simulink library "HEV_Battery_Lib_org"  (Simulink 10.0)
settings: Solver=ode45  StartTime=0.0  StopTime=10.0  RelTol=1e-3  EnableMultiTasking=on
undefined symbols (not defined in the file): HEV_Param, Hydride, Kt_Temps, Metal, Nickel
libraries: fl_lib x55, nesl_utility x30, LeadAcidBattery_lib x12, $bdroot x9, fl_ps_legacy_lib x9, ee_lib x3, powerlib x3, Capacitors_lib x1, electricdrivelib x1
Description:
  | Copyright 2014-2017 The MathWorks, Inc.
settings Model: Creator=smiller  LastModifiedBy=annonymous

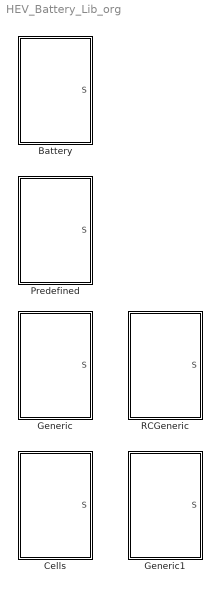
== system HEV_Battery_Lib_org ==
  Battery : Subsystem  BlockChoice=Generic
      settings: TemplateBlock=self  MemberBlocks=Cells,Generic,Predefined
      mask Display: disp(' ')
  Cells : Subsystem
      mask Display:
      | image(imread('HEV_Battery_Cells_IMAGE.jpg'));
      | port_label('LConn',1,'+');
      | port_label('LConn',2,'-');
      | port_label('output',1,'S');
  Generic : Subsystem
      mask Display:
      | image(imread('HEV_Battery_Custom_IMAGE.jpg'));
      | port_label('LConn',1,'+');
      | port_label('LConn',2,'-');
      | port_label('output',1,'S');
  Generic1 : Subsystem
      mask Display:
      | image(imread('HEV_Battery_Generic_IMAGE.jpg'));
      | port_label('LConn',1,'+');
      | port_label('LConn',2,'-');
      | port_label('output',1,'S');
  Predefined : Subsystem
      mask Display:
      | image(imread('HEV_Battery_Detailed_IMAGE.jpg'));
      | port_label('LConn',1,'+');
      | port_label('LConn',2,'-');
      | port_label('output',1,'S');
  RCGeneric : Subsystem
      mask Display:
      | image(imread('HEV_Battery_GenericRC_IMAGE.jpg'));
      | port_label('LConn',1,'+');
      | port_label('LConn',2,'-');
      | port_label('output',1,'S');

== system HEV_Battery_Lib_org/Battery ==
  Generic : $bdroot/Generic  SystemSampleTime=-1  Latency=0  AutoFrameSizeCalculation=off
  + : PMIOPort  Side=Left
  - : PMIOPort  Port=2  Side=Left
  S : Outport
  wires:
  Generic/1 -> S/1
  connections:
  Generic/LConn1 -- +/RConn1
  Generic/LConn2 -- -/RConn1

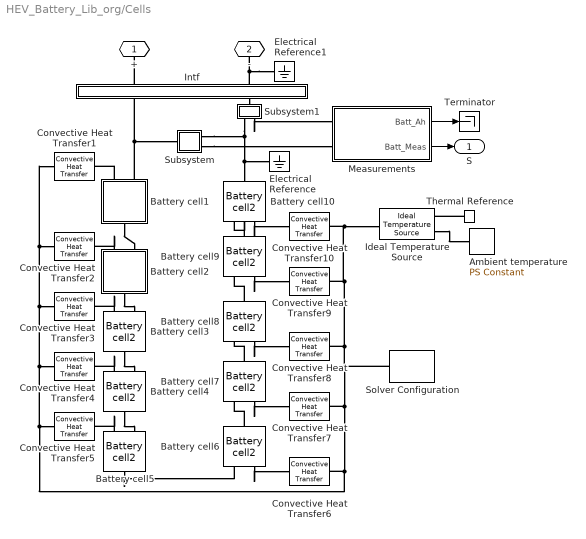
== system HEV_Battery_Lib_org/Cells ==
  Ambient temperature : fl_lib/Physical Signals/Sources/PS Constant  constant=273+25
  Battery cell1 : Subsystem
      mask Display:
      | % Battery icon
      | plot([1.5 0.4],[0 0])
      | plot(-[0.2 0.9 0.9 1.5],[0 0 -0.8 -0.8])
      | patch(([1 1 -1 -1]*0.15-0.5)*-1,[-1 1 1 -1]*0.4,[0;0;0]);
      | patch(([1 1 -1 -1]*0.15+0.1)*-1,[-1 1 1 -1]*0.9,[0;0;0]);
      | 
      | % Thermal port
      | plot([-0.5,-0.9],[1.2,1.2])
      | plot([-0.5,-0.9],[0.4,0.4])
      | plot([-0.9,-1.5],[0.8,0.8])
      | plot(-0.15*sin(0:2*pi/50:2*pi)-0.85,-0.35*cos(0:2*pi/50:2*pi)+0.8)
      | plot(0.15*sin(0:2*pi/50:pi)-0.55,-0.35*cos(0:2*pi/50:pi)+0.8)
      | 
      | % Plot points to set plot range
      | color('white');plot(1.5,1.5);plot(-1.5,-1.5)
      | 
      | color('red')
      | port_label('LConn',1,'H')
      | port_label('LConn',2,'+')
      | port_label('RConn',1,'-')
  Battery cell{3..10} (8 alike) : $bdroot/Cells/Battery cell2  SystemSampleTime=-1
  Battery cell2 : Subsystem
      mask Display:
      | % Battery icon
      | plot([1.5 0.4],[0 0])
      | plot(-[0.2 0.9 0.9 1.5],[0 0 -0.8 -0.8])
      | patch(([1 1 -1 -1]*0.15-0.5)*-1,[-1 1 1 -1]*0.4,[0;0;0]);
      | patch(([1 1 -1 -1]*0.15+0.1)*-1,[-1 1 1 -1]*0.9,[0;0;0]);
      | 
      | % Thermal port
      | plot([-0.5,-0.9],[1.2,1.2])
      | plot([-0.5,-0.9],[0.4,0.4])
      | plot([-0.9,-1.5],[0.8,0.8])
      | plot(-0.15*sin(0:2*pi/50:2*pi)-0.85,-0.35*cos(0:2*pi/50:2*pi)+0.8)
      | plot(0.15*sin(0:2*pi/50:pi)-0.55,-0.35*cos(0:2*pi/50:pi)+0.8)
      | 
      | % Plot points to set plot range
      | color('white');plot(1.5,1.5);plot(-1.5,-1.5)
      | 
      | color('red')
      | port_label('LConn',1,'H')
      | port_label('LConn',2,'+')
      | port_label('RConn',1,'-')
  Convective Heat Transfer{1..10} (10 alike) : fl_lib/Thermal/Thermal Elements/Convective Heat Transfer  area=HEV_Param.Battery_Cell.Area m^2  heat_tr_coeff=HEV_Param.Battery_Cell.Rtheta W/(m^2 *K)  Q_specify=off  Q_priority=High  Q=0 J/s  Q_nominal_specify=off  Q_nominal_unit=J/s  Q_nominal_value=1  T_specify=off  T_priority=High  T=0 K  T_nominal_specify=off  T_nominal_unit=K  T_nominal_value=1
  Electrical Reference : fl_lib/Electrical/Electrical Elements/Electrical Reference
  Electrical Reference1 : fl_lib/Electrical/Electrical Elements/Electrical Reference
  Ideal Temperature Source : fl_lib/Thermal/Thermal Sources/Ideal Temperature Source
      settings: SourceProductName=Simscape  SourceProductBaseCode=SS
  Intf : Subsystem  mask(Simscape Interface Element){T=100000}
      mask prompts: T "Pole in Transfer Function"
      mask help:
      | Ideal transformer between Simscape circuits.
      |
      | The Voltage across the two terminal pairs are equal and the current flowing through the two branches are equal.
      |
      | The coupling has a transfer function and you need to set the pole in the transfer function.
      mask Display:
      | %color('red');
      | %plot([0.3 0.7],[0.775 0.775]);
      | port_label('LConn', 1,'SPS1')
      | port_label('RConn', 1,'SS1')
      | color('black');
      | %plot([0.3 0.7],[0.225 0.225]);
      | port_label('LConn', 2,'SPS2')
      | port_label('RConn', 2,'SS2')
      | color('green')
      | %text(0.05,0.5,'I Src');
      | color('blue')
      | %text(0.75,0.5,'V Src');
  Measurements : Subsystem
  Solver Configuration : nesl_utility/Solver Configuration  PhysicalDomain=network_engine_domain  SubClassName=solver  LeftPortType=input  RightPortType=generic  Accelerate=off  Tones=[]  Harmonics=[]  SimulateNoise=off  Profile=off  UseLocalSampling=off  EnableSwitchedLinearOptims=on  FrequencyDomain=off  UseCCode=off  RelTol=0.001  AbsTol=1e-06  MinStep=1e-09  ToWorkspace=off  RevertToSquareIcSolve=off  NumHomotopyIterations=100  PhasorMode=off  PhasorModeNumHarmonics=1  OverrideAbsTol=off  DoDC=off  ResidualTolerance=1e-9  UseLocalSolver=off  LocalSolverChoice=NE_BACKWARD_EULER_ADVANCER  LocalSolverSampleTime=.001  DoFixedCost=off  MaxNonlinIter=3  MaxModeIter=2  LinearAlgebra=Sparse  DelaysMemoryBudget=1024  AutomaticFiltering=on  FilteringTimeConstant=0.001
  Subsystem : Subsystem
      mask Display: disp('S')
  Subsystem1 : Subsystem
      mask Display: disp('S');
  Terminator : Terminator
  Thermal Reference : fl_lib/Thermal/Thermal Elements/Thermal Reference
  + : PMIOPort  Side=Left
  - : PMIOPort  Port=2  Side=Left
  S : Outport
  wires:
  Measurements/2(Batt_Meas) -> S/1
  Measurements/1(Batt_Ah) -> Terminator/1
  connections:
  Electrical Reference1/LConn1 -- -/RConn1 -- Intf/RConn2
  Intf/RConn1 -- +/RConn1
  Intf/LConn2 -- Subsystem1/LConn1
  Subsystem1/RConn2 -- Measurements/LConn1
  Subsystem1/RConn1 -- Battery cell10/RConn1 -- Electrical Reference/LConn1 -- Subsystem/RConn2
  Subsystem/RConn1 -- Measurements/LConn2
  Convective Heat Transfer6/LConn1 -- Convective Heat Transfer1/LConn1 -- Convective Heat Transfer2/LConn1 -- Convective Heat Transfer3/LConn1 -- Convective Heat Transfer4/LConn1 -- Convective Heat Transfer5/LConn1 -- Solver Configuration/RConn1 -- Convective Heat Transfer8/LConn1 -- Convective Heat Transfer10/LConn1 -- Ideal Temperature Source/LConn1 -- Convective Heat Transfer9/LConn1 -- Convective Heat Transfer7/LConn1
  Battery cell1/LConn2 -- Subsystem/LConn1 -- Intf/LConn1
  Battery cell9/LConn1 -- Convective Heat Transfer9/RConn1
  Battery cell8/RConn1 -- Battery cell9/LConn2
  Battery cell8/LConn1 -- Convective Heat Transfer8/RConn1
  Battery cell7/LConn1 -- Convective Heat Transfer7/RConn1
  Battery cell7/RConn1 -- Battery cell8/LConn2
  Battery cell6/LConn1 -- Convective Heat Transfer6/RConn1
  Battery cell6/RConn1 -- Battery cell7/LConn2
  Battery cell5/RConn1 -- Battery cell6/LConn2
  Battery cell5/LConn1 -- Convective Heat Transfer5/RConn1
  Battery cell4/RConn1 -- Battery cell5/LConn2
  Battery cell4/LConn1 -- Convective Heat Transfer4/RConn1
  Battery cell3/RConn1 -- Battery cell4/LConn2
  Battery cell3/LConn1 -- Convective Heat Transfer3/RConn1
  Battery cell2/RConn1 -- Battery cell3/LConn2
  Battery cell9/RConn1 -- Battery cell10/LConn2
  Battery cell2/LConn1 -- Convective Heat Transfer2/RConn1
  Battery cell10/LConn1 -- Convective Heat Transfer10/RConn1
  Battery cell1/RConn1 -- Battery cell2/LConn2
  Battery cell1/LConn1 -- Convective Heat Transfer1/RConn1
  Ideal Temperature Source/RConn1 -- Ambient temperature/RConn1
  Thermal Reference/LConn1 -- Ideal Temperature Source/RConn2

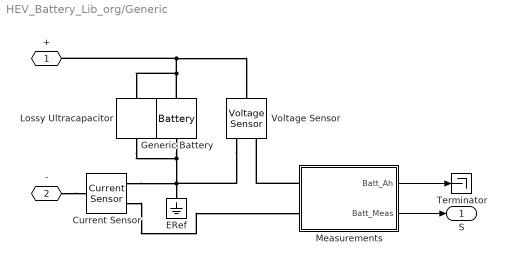
== system HEV_Battery_Lib_org/Generic ==
  Current Sensor : fl_lib/Electrical/Electrical Sensors/Current Sensor
  ERef : fl_lib/Electrical/Electrical Elements/Electrical Reference
  Generic Battery : ee_lib/Sources/Battery  Vnom=HEV_Param.Battery_Sys.Nominal_Voltage V  R1=HEV_Param.Battery_Sys.Internal_Resistance Ohm  prm_AH=2  AH=HEV_Param.Battery_Sys.Rated_Capacity hr*A  V1=HEV_Param.Battery_Sys.Expn_Voltage V  AH1=HEV_Param.Battery_Sys.Expn_Charge hr*A  prm_R2=1  R2=2e+3 Ohm  prm_dyn=1  Rp1=0.005 Ohm  tau1=30 s  Rp2=0.005 Ohm  tau2=30 s  Rp3=0.005 Ohm  tau3=30 s  Rp4=0.005 Ohm  tau4=30 s  Rp5=0.005 Ohm  tau5=30 s  prm_fade=1  N_fade=100  AH_fade=45 hr*A  R1_fade=2.02 Ohm  V1_fade=10.35 V  i_specify=off  i_priority=None  i=0 A  i_nominal_specify=off  i_nominal_unit=A  i_nominal_value=1  v_specify=off  v_priority=None  v=0 V  v_nominal_specify=off  v_nominal_unit=V  v_nominal_value=1  charge_specify=on  charge_priority=High  charge=HEV_Param.Battery_Sys.Initial_Charge hr*A  charge_nominal_specify=off  charge_nominal_unit=hr*A  charge_nominal_value=1  num_cycles_specify=off  num_cycles_priority=High  num_cycles=0  num_cycles_nominal_specify=off  num_cycles_nominal_unit=1  num_cycles_nominal_value=1  thermal_mass=30000 J/K  Tmeas=298.15 K  Vnom_T2=12 V  R1_T2=2.2 Ohm  V1_T2=11.4 V  R2_T2=2200 Ohm  Rp1_T2=0.005 Ohm  tau1_T2=30 s  Rp2_T2=0.005 Ohm  tau2_T2=30 s  Rp3_T2=0.005 Ohm  tau3_T2=30 s  Rp4_T2=0.005 Ohm  tau4_T2=30 s  Rp5_T2=0.005 Ohm  tau5_T2=30 s  Tmeas2=273.15 K  temperature_specify=off  temperature_priority=High  temperature=298.15 K  temperature_nominal_specify=off  temperature_nominal_unit=K  temperature_nominal_value=1
      settings: SourceProductName=Simscape Electrical
  Lossy Ultracapacitor : Capacitors_lib/Lossy Ultracapacitor  C0=HEV_Param.UltraCapacitor.Nominal_Capacitance F  Cv=HEV_Param.UltraCapacitor.Rate_C_V F/V  R=HEV_Param.UltraCapacitor.Series_R Ohm  Rd=HEV_Param.UltraCapacitor.Self_Discharge_R Ohm  i_specify=off  i_priority=High  i=0 A  i_nominal_specify=off  i_nominal_unit=A  i_nominal_value=1  vc_specify=off  vc_priority=High  vc=0 V  vc_nominal_specify=off  vc_nominal_unit=V  vc_nominal_value=1
      settings: InternalSimscapePortConfiguration="{\"Bottom\":[],\"Left\":[{\"id\":\"p\",\"label\":\"+\",\"type\":\"foundation.electrical.electrical\"}],\"Right\":[{\"id\":\"n\",\"label\":\"-\",\"type\":\"foundation.electrical.electrical\"}],\"Top\":[]}"
  Measurements : Subsystem
  Terminator : Terminator
  Voltage Sensor : fl_lib/Electrical/Electrical Sensors/Voltage Sensor
  + : PMIOPort  Side=Left
  - : PMIOPort  Port=2  Side=Left
  S : Outport
  wires:
  Measurements/1(Batt_Ah) -> Terminator/1
  Measurements/2(Batt_Meas) -> S/1
  connections:
  Measurements/LConn1 -- Voltage Sensor/RConn1
  Generic Battery/LConn1 -- Voltage Sensor/LConn1 -- +/RConn1 -- Lossy Ultracapacitor/LConn1
  Generic Battery/RConn1 -- Voltage Sensor/RConn2 -- ERef/LConn1 -- Current Sensor/RConn2 -- Lossy Ultracapacitor/RConn1
  Current Sensor/RConn1 -- Measurements/LConn2
  -/RConn1 -- Current Sensor/LConn1

== system HEV_Battery_Lib_org/Generic1 ==
  Current Sensor : fl_lib/Electrical/Electrical Sensors/Current Sensor
  Electrical Reference : fl_lib/Electrical/Electrical Elements/Electrical Reference
  Generic Battery : ee_lib/Sources/Battery  Vnom=HEV_Param.Battery_Sys.Nominal_Voltage V  R1=HEV_Param.Battery_Sys.Internal_Resistance Ohm  prm_AH=2  AH=HEV_Param.Battery_Sys.Rated_Capacity hr*A  V1=HEV_Param.Battery_Sys.Expn_Voltage V  AH1=HEV_Param.Battery_Sys.Expn_Charge hr*A  prm_R2=1  R2=2e+3 Ohm  prm_dyn=1  Rp1=0.005 Ohm  tau1=30 s  Rp2=0.005 Ohm  tau2=30 s  Rp3=0.005 Ohm  tau3=30 s  Rp4=0.005 Ohm  tau4=30 s  Rp5=0.005 Ohm  tau5=30 s  prm_fade=1  N_fade=100  AH_fade=45 hr*A  R1_fade=2.02 Ohm  V1_fade=10.35 V  i_specify=off  i_priority=None  i=0 A  i_nominal_specify=off  i_nominal_unit=A  i_nominal_value=1  v_specify=off  v_priority=None  v=0 V  v_nominal_specify=off  v_nominal_unit=V  v_nominal_value=1  charge_specify=on  charge_priority=High  charge=HEV_Param.Battery_Sys.Initial_Charge hr*A  charge_nominal_specify=off  charge_nominal_unit=hr*A  charge_nominal_value=1  num_cycles_specify=off  num_cycles_priority=High  num_cycles=0  num_cycles_nominal_specify=off  num_cycles_nominal_unit=1  num_cycles_nominal_value=1  thermal_mass=30000 J/K  Tmeas=298.15 K  Vnom_T2=12 V  R1_T2=2.2 Ohm  V1_T2=11.4 V  R2_T2=2200 Ohm  Rp1_T2=0.005 Ohm  tau1_T2=30 s  Rp2_T2=0.005 Ohm  tau2_T2=30 s  Rp3_T2=0.005 Ohm  tau3_T2=30 s  Rp4_T2=0.005 Ohm  tau4_T2=30 s  Rp5_T2=0.005 Ohm  tau5_T2=30 s  Tmeas2=273.15 K  temperature_specify=off  temperature_priority=High  temperature=298.15 K  temperature_nominal_specify=off  temperature_nominal_unit=K  temperature_nominal_value=1
      settings: SourceProductName=Simscape Electrical
  Measurements : Subsystem
  Terminator : Terminator
  Voltage Sensor1 : fl_lib/Electrical/Electrical Sensors/Voltage Sensor
  + : PMIOPort  Side=Left
  - : PMIOPort  Port=2  Side=Left
  S : Outport
  wires:
  Measurements/2(Batt_Meas) -> S/1
  Measurements/1(Batt_Ah) -> Terminator/1
  connections:
  -/RConn1 -- Current Sensor/LConn1
  Current Sensor/RConn1 -- Measurements/LConn2
  Current Sensor/RConn2 -- Electrical Reference/LConn1 -- Generic Battery/RConn1 -- Voltage Sensor1/RConn2
  +/RConn1 -- Generic Battery/LConn1 -- Voltage Sensor1/LConn1
  Measurements/LConn1 -- Voltage Sensor1/RConn1

== system HEV_Battery_Lib_org/Predefined ==
  Electrical Reference : fl_lib/Electrical/Electrical Elements/Electrical Reference
  GF1 : Subsystem
      mask Display: disp('GF')
  Ground : powerlib/Elements/Ground  LConnTagsString=a
      settings: SourceProductName=Simscape Electrical
  Intf : Subsystem  mask(Power Systems ST - Simscape Interface Element){T=100000}
      mask prompts: T "Pole in Transfer Function"
      mask help:
      | Ideal transformer between a Simscape Power Systems ST circuit and a Simscape circuit.
      |
      | The Voltage across the two terminal pairs are equal and the current flowing through the two branches are equal.
      |
      | The coupling has a transfer function and you need to set the pole in the transfer function.
      mask Display:
      | %color('red');
      | %plot([0.3 0.7],[0.775 0.775]);
      | port_label('LConn', 1,'SPS1')
      | port_label('RConn', 1,'SS1')
      | color('black');
      | %plot([0.3 0.7],[0.225 0.225]);
      | port_label('LConn', 2,'SPS2')
      | port_label('RConn', 2,'SS2')
      | color('green')
      | %text(0.05,0.5,'I Src');
      | color('blue')
      | %text(0.75,0.5,'V Src');
  Preset Battery : electricdrivelib/Extra Sources/Battery  BatType=Nickel-Metal-Hydride  ShowTempParam=off  ThermalPreset=no  ShowAgeParam=off  NomV=HEV_Param.Battery_Det.Nominal_Voltage  NomQ=HEV_Param.Battery_Det.Rated_Capacity  SOC=HEV_Param.Battery_Det.Initial_SOC  Batt_Tr=30  PresetModel=on  MaxQ=8.7231  MinV=150  FullV=235.5932  Dis_rate=1.62  R=0.24691  Normal_OP=7.7885  expZone="[216.9492          1.62]"  current=[50 100]  Units=Time  Tci=20  NomT=20  T2=-30  MaxQ2=4.8  FullV2=7.1  Normal_OP2=5.72  expZone2="[6.58  1]"  Rca=0.6  ti=1000  Dp=0  Neq0=0  Tsim=1e6  Ta1=25  Qeol=5.4*0.9  Reol=0.013333*1.2  Char_age=[2.3478, 3]  Dis_age=[2.3478, 10]  N1=1500  N2=10500  N3=1000  N4=1400  Ta2=45  N5=950
      settings: SourceProductName=Simscape Electrical
  + : PMIOPort  Side=Left
  - : PMIOPort  Port=2  Side=Left
  S : Outport
  wires:
  Preset Battery/1 -> GF1/1(In1)
  GF1/1(Out1) -> S/1
  connections:
  Intf/RConn2 -- Electrical Reference/LConn1 -- -/RConn1
  Intf/LConn2 -- Ground/LConn1 -- Preset Battery/LConn2
  Preset Battery/LConn1 -- Intf/LConn1
  +/RConn1 -- Intf/RConn1

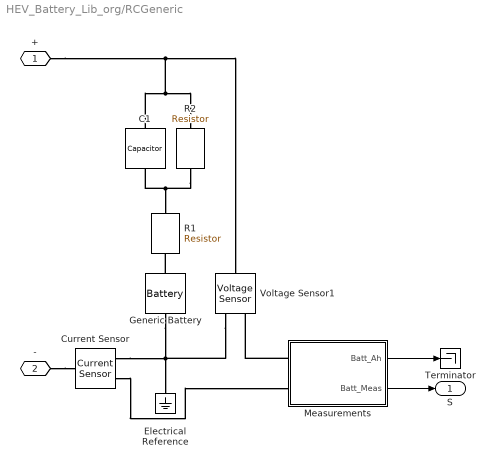
== system HEV_Battery_Lib_org/RCGeneric ==
  C1 : fl_lib/Electrical/Electrical Elements/Capacitor  c=HEV_Param.Battery_Sys.C1.Capacitance F  r=HEV_Param.Battery_Sys.C1.Series_Resistance Ohm  g=0 1/Ohm  i_specify=off  i_priority=High  i=0 A  i_nominal_specify=off  i_nominal_unit=A  i_nominal_value=1  v_specify=off  v_priority=High  v=0 V  v_nominal_specify=off  v_nominal_unit=V  v_nominal_value=1  vc_specify=on  vc_priority=High  vc=HEV_Param.Battery_Sys.C1.Initial_Voltage V  vc_nominal_specify=off  vc_nominal_unit=V  vc_nominal_value=1
  Current Sensor : fl_lib/Electrical/Electrical Sensors/Current Sensor
  Electrical Reference : fl_lib/Electrical/Electrical Elements/Electrical Reference
  Generic Battery : ee_lib/Sources/Battery  Vnom=HEV_Param.Battery_Sys.Nominal_Voltage V  R1=HEV_Param.Battery_Sys.Internal_Resistance Ohm  prm_AH=2  AH=HEV_Param.Battery_Sys.Rated_Capacity hr*A  V1=HEV_Param.Battery_Sys.Expn_Voltage V  AH1=HEV_Param.Battery_Sys.Expn_Charge hr*A  prm_R2=1  R2=2e+3 Ohm  prm_dyn=1  Rp1=0.005 Ohm  tau1=30 s  Rp2=0.005 Ohm  tau2=30 s  Rp3=0.005 Ohm  tau3=30 s  Rp4=0.005 Ohm  tau4=30 s  Rp5=0.005 Ohm  tau5=30 s  prm_fade=1  N_fade=100  AH_fade=45 hr*A  R1_fade=2.02 Ohm  V1_fade=10.35 V  i_specify=off  i_priority=None  i=0 A  i_nominal_specify=off  i_nominal_unit=A  i_nominal_value=1  v_specify=off  v_priority=None  v=0 V  v_nominal_specify=off  v_nominal_unit=V  v_nominal_value=1  charge_specify=on  charge_priority=High  charge=HEV_Param.Battery_Sys.Initial_Charge hr*A  charge_nominal_specify=off  charge_nominal_unit=hr*A  charge_nominal_value=1  num_cycles_specify=off  num_cycles_priority=High  num_cycles=0  num_cycles_nominal_specify=off  num_cycles_nominal_unit=1  num_cycles_nominal_value=1  thermal_mass=30000 J/K  Tmeas=298.15 K  Vnom_T2=12 V  R1_T2=2.2 Ohm  V1_T2=11.4 V  R2_T2=2200 Ohm  Rp1_T2=0.005 Ohm  tau1_T2=30 s  Rp2_T2=0.005 Ohm  tau2_T2=30 s  Rp3_T2=0.005 Ohm  tau3_T2=30 s  Rp4_T2=0.005 Ohm  tau4_T2=30 s  Rp5_T2=0.005 Ohm  tau5_T2=30 s  Tmeas2=273.15 K  temperature_specify=off  temperature_priority=High  temperature=298.15 K  temperature_nominal_specify=off  temperature_nominal_unit=K  temperature_nominal_value=1
      settings: SourceProductName=Simscape Electrical
  Measurements : Subsystem
  R1 : fl_lib/Electrical/Electrical Elements/Resistor  R=HEV_Param.Battery_Sys.R1 Ohm  i_specify=off  i_priority=High  i=0 A  i_nominal_specify=off  i_nominal_unit=A  i_nominal_value=1  v_specify=off  v_priority=High  v=0 V  v_nominal_specify=off  v_nominal_unit=V  v_nominal_value=1
  R2 : fl_lib/Electrical/Electrical Elements/Resistor  R=HEV_Param.Battery_Sys.R2 Ohm  i_specify=off  i_priority=High  i=0 A  i_nominal_specify=off  i_nominal_unit=A  i_nominal_value=1  v_specify=off  v_priority=High  v=0 V  v_nominal_specify=off  v_nominal_unit=V  v_nominal_value=1
  Terminator : Terminator
  Voltage Sensor1 : fl_lib/Electrical/Electrical Sensors/Voltage Sensor
  + : PMIOPort  Side=Left
  - : PMIOPort  Port=2  Side=Left
  S : Outport
  wires:
  Measurements/1(Batt_Ah) -> Terminator/1
  Measurements/2(Batt_Meas) -> S/1
  connections:
  Measurements/LConn1 -- Voltage Sensor1/RConn1
  +/RConn1 -- Voltage Sensor1/LConn1 -- R2/LConn1 -- C1/LConn1
  Voltage Sensor1/RConn2 -- Generic Battery/RConn1 -- Electrical Reference/LConn1 -- Current Sensor/RConn2
  Current Sensor/RConn1 -- Measurements/LConn2
  -/RConn1 -- Current Sensor/LConn1
  R2/RConn1 -- R1/LConn1 -- C1/RConn1
  Generic Battery/LConn1 -- R1/RConn1

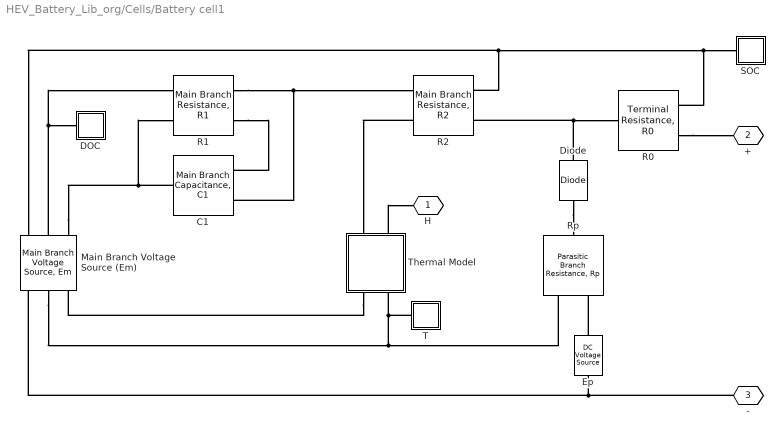
== system HEV_Battery_Lib_org/Cells/Battery cell1 ==
  " DOC " : Subsystem
  " SOC " : Subsystem
  C1 : LeadAcidBattery_lib/Main Branch Capacitance, C1  Tau1=HEV_Param.Battery_Cell.Tau1 s  Cmin=1e-5 F
  Diode : fl_lib/Electrical/Electrical Elements/Diode  Vf=0.6 V  Ron=0.3 Ohm  Goff=1e-08 1/Ohm  i_specify=off  i_priority=High  i=0 A  i_nominal_specify=off  i_nominal_unit=A  i_nominal_value=1  v_specify=off  v_priority=High  v=0 V  v_nominal_specify=off  v_nominal_unit=V  v_nominal_value=1
  Ep : fl_lib/Electrical/Electrical Sources/DC Voltage Source  v0=HEV_Param.Battery_Cell.Ep V
  Main Branch Voltage Source (Em) : LeadAcidBattery_lib/Main Branch Voltage Source, Em  Em0=HEV_Param.Battery_Cell.Emo V  Ke=HEV_Param.Battery_Cell.Ke V/K  Kc=HEV_Param.Battery_Cell.Kc  C0=HEV_Param.Battery_Cell.Costar s*A  Istar=HEV_Param.Battery_Cell.Istar A  delta=HEV_Param.Battery_Cell.delta  Tau1=HEV_Param.Battery_Cell.Tau1 s  Qinit=HEV_Param.Battery_Cell.Qe_init s*A
  R0 : LeadAcidBattery_lib/Terminal Resistance, R0  R00=HEV_Param.Battery_Cell.Roo Ohm  A0=HEV_Param.Battery_Cell.Ao
  R1 : LeadAcidBattery_lib/Main Branch Resistance, R1  R10=HEV_Param.Battery_Cell.R10 Ohm  DOC_min=1e-006
  R2 : LeadAcidBattery_lib/Main Branch Resistance, R2  R20=HEV_Param.Battery_Cell.R20 Ohm  A21=HEV_Param.Battery_Cell.A21  A22=HEV_Param.Battery_Cell.A22  Istar=HEV_Param.Battery_Cell.Istar A
  Rp : LeadAcidBattery_lib/Parasitic Branch Resistance, Rp  Gp0=HEV_Param.Battery_Cell.Gpo 1/Ohm  Vp0=HEV_Param.Battery_Cell.Vpo V  Ap=HEV_Param.Battery_Cell.Ap  Tf=HEV_Param.Battery_Cell.theta_f degC
  T : Subsystem
  Thermal Model : Subsystem
  H : PMIOPort  Tag=PMCPort  Side=Left
  + : PMIOPort  Tag=PMCPort  Port=2  Side=Left
  - : PMIOPort  Tag=PMCPort  Port=3  Side=Right
  connections:
  Diode/LConn1 -- R0/RConn1 -- R2/LConn2
  R2/RConn2 -- Thermal Model/LConn1
  -/RConn1 -- Ep/RConn1 -- Main Branch Voltage Source (Em)/RConn1
  Thermal Model/RConn1 -- Main Branch Voltage Source (Em)/RConn3
  Diode/RConn1 -- Rp/LConn1
  Ep/LConn1 -- Rp/RConn2
  Thermal Model/LConn2 -- H/RConn1
  R2/LConn1 -- Main Branch Voltage Source (Em)/LConn1 -- R0/LConn1 -- " SOC "/LConn1
  R1/LConn2 -- C1/LConn1
  R1/LConn1 -- C1/LConn2 -- R2/RConn1
  Main Branch Voltage Source (Em)/LConn3 -- C1/RConn1 -- R1/RConn2
  Main Branch Voltage Source (Em)/LConn2 -- R1/RConn1 -- " DOC "/LConn1
  R0/LConn2 -- +/RConn1
  Main Branch Voltage Source (Em)/RConn2 -- Rp/RConn1 -- T/LConn1 -- Thermal Model/RConn2

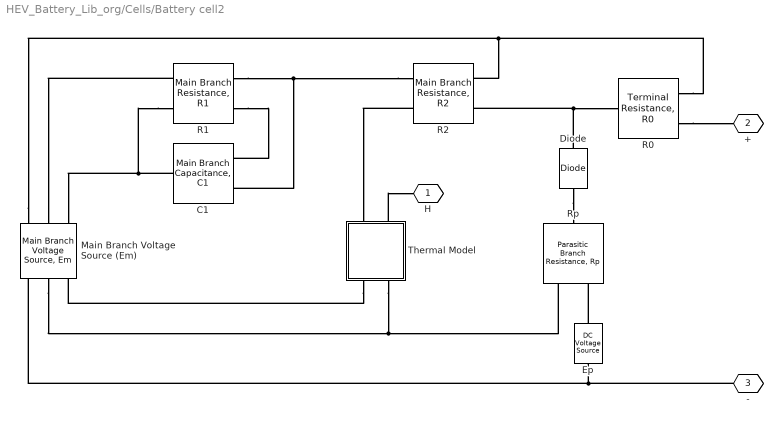
== system HEV_Battery_Lib_org/Cells/Battery cell2 ==
  C1 : LeadAcidBattery_lib/Main Branch Capacitance, C1  Tau1=HEV_Param.Battery_Cell.Tau1 s  Cmin=1e-5 F
  Diode : fl_lib/Electrical/Electrical Elements/Diode  Vf=0.6 V  Ron=0.3 Ohm  Goff=1e-08 1/Ohm  i_specify=off  i_priority=High  i=0 A  i_nominal_specify=off  i_nominal_unit=A  i_nominal_value=1  v_specify=off  v_priority=High  v=0 V  v_nominal_specify=off  v_nominal_unit=V  v_nominal_value=1
  Ep : fl_lib/Electrical/Electrical Sources/DC Voltage Source  v0=HEV_Param.Battery_Cell.Ep V
  Main Branch Voltage Source (Em) : LeadAcidBattery_lib/Main Branch Voltage Source, Em  Em0=HEV_Param.Battery_Cell.Emo V  Ke=HEV_Param.Battery_Cell.Ke V/K  Kc=HEV_Param.Battery_Cell.Kc  C0=HEV_Param.Battery_Cell.Costar s*A  Istar=HEV_Param.Battery_Cell.Istar A  delta=HEV_Param.Battery_Cell.delta  Tau1=HEV_Param.Battery_Cell.Tau1 s  Qinit=HEV_Param.Battery_Cell.Qe_init s*A
  R0 : LeadAcidBattery_lib/Terminal Resistance, R0  R00=HEV_Param.Battery_Cell.Roo Ohm  A0=HEV_Param.Battery_Cell.Ao
  R1 : LeadAcidBattery_lib/Main Branch Resistance, R1  R10=HEV_Param.Battery_Cell.R10 Ohm  DOC_min=1e-006
  R2 : LeadAcidBattery_lib/Main Branch Resistance, R2  R20=HEV_Param.Battery_Cell.R20 Ohm  A21=HEV_Param.Battery_Cell.A21  A22=HEV_Param.Battery_Cell.A22  Istar=HEV_Param.Battery_Cell.Istar A
  Rp : LeadAcidBattery_lib/Parasitic Branch Resistance, Rp  Gp0=HEV_Param.Battery_Cell.Gpo 1/Ohm  Vp0=HEV_Param.Battery_Cell.Vpo V  Ap=HEV_Param.Battery_Cell.Ap  Tf=HEV_Param.Battery_Cell.theta_f degC
  Thermal Model : Subsystem
  H : PMIOPort  Tag=PMCPort  Side=Left
  + : PMIOPort  Tag=PMCPort  Port=2  Side=Left
  - : PMIOPort  Tag=PMCPort  Port=3  Side=Right
  connections:
  Rp/RConn1 -- Main Branch Voltage Source (Em)/RConn2 -- Thermal Model/RConn2
  R0/LConn2 -- +/RConn1
  R1/RConn1 -- Main Branch Voltage Source (Em)/LConn2
  R1/RConn2 -- C1/RConn1 -- Main Branch Voltage Source (Em)/LConn3
  R2/RConn1 -- C1/LConn2 -- R1/LConn1
  R1/LConn2 -- C1/LConn1
  Main Branch Voltage Source (Em)/LConn1 -- R2/LConn1 -- R0/LConn1
  Thermal Model/LConn2 -- H/RConn1
  Ep/LConn1 -- Rp/RConn2
  Diode/RConn1 -- Rp/LConn1
  Thermal Model/RConn1 -- Main Branch Voltage Source (Em)/RConn3
  Main Branch Voltage Source (Em)/RConn1 -- Ep/RConn1 -- -/RConn1
  R2/RConn2 -- Thermal Model/LConn1
  R2/LConn2 -- R0/RConn1 -- Diode/LConn1

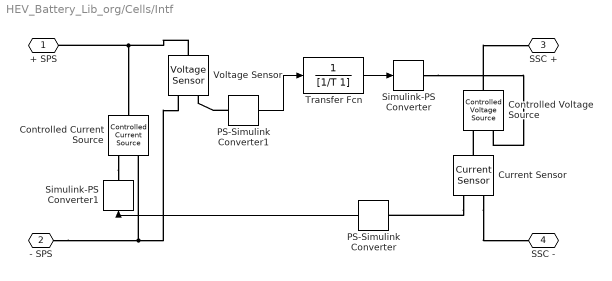
== system HEV_Battery_Lib_org/Cells/Intf ==
  Controlled Voltage Source : fl_lib/Electrical/Electrical Sources/Controlled Voltage Source
  Controlled Current Source : fl_lib/Electrical/Electrical Sources/Controlled Current Source
  Current Sensor : fl_lib/Electrical/Electrical Sensors/Current Sensor
  PS-Simulink Converter : nesl_utility/PS-Simulink Converter  PhysicalDomain=network_engine_domain  SubClassName=ps_output  LeftPortType=input  RightPortType=output  PseudoPeriodic=off  Frequencies=[]  Unit=A  AffineConversion=off
  PS-Simulink Converter1 : nesl_utility/PS-Simulink Converter  PhysicalDomain=network_engine_domain  SubClassName=ps_output  LeftPortType=input  RightPortType=output  PseudoPeriodic=off  Frequencies=[]  Unit=V  AffineConversion=off
  Simulink-PS Converter : nesl_utility/Simulink-PS Converter  PhysicalDomain=network_engine_domain  SubClassName=ps_input  LeftPortType=input  RightPortType=output  PseudoPeriodic=off  Frequencies=[]  NoiseDistribution=none  NoiseParameters=[]  Unit=V  AffineConversion=off  FilteringAndDerivatives=zero  SimscapeFilterOrder=1  InputFilterTimeConstant=.001  UdotUserProvided=0
  Simulink-PS Converter1 : nesl_utility/Simulink-PS Converter  PhysicalDomain=network_engine_domain  SubClassName=ps_input  LeftPortType=input  RightPortType=output  PseudoPeriodic=off  Frequencies=[]  NoiseDistribution=none  NoiseParameters=[]  Unit=A  AffineConversion=off  FilteringAndDerivatives=zero  SimscapeFilterOrder=1  InputFilterTimeConstant=.001  UdotUserProvided=0
  Transfer Fcn : TransferFcn  Denominator=[1/T 1]
  Voltage Sensor : fl_lib/Electrical/Electrical Sensors/Voltage Sensor
  + SPS : PMIOPort  Side=Left
  - SPS : PMIOPort  Port=2  Side=Left
  SSC + : PMIOPort  Port=3  Side=Right
  SSC - : PMIOPort  Port=4  Side=Right
  wires:
  PS-Simulink Converter1/1 -> Transfer Fcn/1
  Transfer Fcn/1 -> Simulink-PS Converter/1
  PS-Simulink Converter/1 -> Simulink-PS Converter1/1
  connections:
  Controlled Current Source/RConn1 -- Simulink-PS Converter1/RConn1
  PS-Simulink Converter1/LConn1 -- Voltage Sensor/RConn1
  Voltage Sensor/LConn1 -- + SPS/RConn1 -- Controlled Current Source/LConn1
  Current Sensor/RConn2 -- SSC -/RConn1
  Voltage Sensor/RConn2 -- - SPS/RConn1 -- Controlled Current Source/RConn2
  Current Sensor/RConn1 -- PS-Simulink Converter/LConn1
  Simulink-PS Converter/RConn1 -- Controlled Voltage Source/RConn1
  Current Sensor/LConn1 -- Controlled Voltage Source/RConn2
  Controlled Voltage Source/LConn1 -- SSC +/RConn1

== system HEV_Battery_Lib_org/Cells/Measurements ==
  Bus Creator : BusCreator  Inputs=4
  Calc Pct : Gain  Gain=1/HEV_Param.Battery_Sys.Maximum_Capacity*100
  Calculate battery power & charge : Subsystem
  PS-Simulink Converter1 : nesl_utility/PS-Simulink Converter  PhysicalDomain=network_engine_domain  SubClassName=ps_output  LeftPortType=input  RightPortType=output  PseudoPeriodic=off  Frequencies=[]  Unit=V  AffineConversion=off
  PS-Simulink Converter2 : nesl_utility/PS-Simulink Converter  PhysicalDomain=network_engine_domain  SubClassName=ps_output  LeftPortType=input  RightPortType=output  PseudoPeriodic=off  Frequencies=[]  Unit=A  AffineConversion=off
  IBatt : PMIOPort  Side=Left
  VBatt : PMIOPort  Port=2  Side=Left
  Batt_Ah : Outport
  Batt_Meas : Outport  Port=2
  tag scope: Batt_Measures=global
  wires:
  Bus Creator/1 -> Batt_Meas/1, [Batt_Measures]
  PS-Simulink Converter2/1 -> Bus Creator/4  "Current (A)"
  PS-Simulink Converter1/1 -> Bus Creator/3  "Voltage (V)"
  Calc Pct/1 -> Bus Creator/2  "SOC (%)"
  Calculate battery power & charge/1(Ah) -> Batt_Ah/1, Calc Pct/1, Bus Creator/1  "Batt_Ah"
  connections:
  PS-Simulink Converter2/LConn1 -- IBatt/RConn1 -- Calculate battery power & charge/LConn2
  PS-Simulink Converter1/LConn1 -- VBatt/RConn1 -- Calculate battery power & charge/LConn1

== system HEV_Battery_Lib_org/Cells/Subsystem ==
  Voltage Sensor1 : fl_lib/Electrical/Electrical Sensors/Voltage Sensor
  Conn1 : PMIOPort  Side=Right
  Conn2 : PMIOPort  Port=2  Side=Left
  Conn3 : PMIOPort  Port=3  Side=Right
  connections:
  Conn3/RConn1 -- Voltage Sensor1/RConn2
  Conn2/RConn1 -- Voltage Sensor1/LConn1
  Conn1/RConn1 -- Voltage Sensor1/RConn1

== system HEV_Battery_Lib_org/Cells/Subsystem1 ==
  Current Sensor : fl_lib/Electrical/Electrical Sensors/Current Sensor
  Conn1 : PMIOPort  Side=Left
  Conn3 : PMIOPort  Port=2  Side=Right
  Conn2 : PMIOPort  Port=3  Side=Right
  connections:
  Conn3/RConn1 -- Current Sensor/RConn2
  Conn2/RConn1 -- Current Sensor/RConn1
  Conn1/RConn1 -- Current Sensor/LConn1

== system HEV_Battery_Lib_org/Generic/Measurements ==
  Bus Creator : BusCreator  Inputs=4
  Calc Pct : Gain  Gain=1/HEV_Param.Battery_Sys.Maximum_Capacity*100
  Calculate battery power & charge : Subsystem
  PS-Simulink Converter1 : nesl_utility/PS-Simulink Converter  PhysicalDomain=network_engine_domain  SubClassName=ps_output  LeftPortType=input  RightPortType=output  PseudoPeriodic=off  Frequencies=[]  Unit=V  AffineConversion=off
  PS-Simulink Converter2 : nesl_utility/PS-Simulink Converter  PhysicalDomain=network_engine_domain  SubClassName=ps_output  LeftPortType=input  RightPortType=output  PseudoPeriodic=off  Frequencies=[]  Unit=A  AffineConversion=off
  VBatt : PMIOPort  Side=Left
  IBatt : PMIOPort  Port=2  Side=Left
  Batt_Ah : Outport
  Batt_Meas : Outport  Port=2
  tag scope: Batt_Measures=global
  wires:
  Bus Creator/1 -> Batt_Meas/1, [Batt_Measures]
  PS-Simulink Converter2/1 -> Bus Creator/4  "Current (A)"
  PS-Simulink Converter1/1 -> Bus Creator/3  "Voltage (V)"
  Calc Pct/1 -> Bus Creator/2  "SOC (%)"
  Calculate battery power & charge/1(Ah) -> Batt_Ah/1, Calc Pct/1, Bus Creator/1  "Batt_Ah"
  connections:
  PS-Simulink Converter2/LConn1 -- IBatt/RConn1 -- Calculate battery power & charge/LConn2
  PS-Simulink Converter1/LConn1 -- VBatt/RConn1 -- Calculate battery power & charge/LConn1

== system HEV_Battery_Lib_org/Generic1/Measurements ==
  Bus Creator : BusCreator  Inputs=4
  Calc Pct : Gain  Gain=1/HEV_Param.Battery_Sys.Maximum_Capacity*100
  Calculate battery power & charge : Subsystem
  PS-Simulink Converter1 : nesl_utility/PS-Simulink Converter  PhysicalDomain=network_engine_domain  SubClassName=ps_output  LeftPortType=input  RightPortType=output  PseudoPeriodic=off  Frequencies=[]  Unit=V  AffineConversion=off
  PS-Simulink Converter2 : nesl_utility/PS-Simulink Converter  PhysicalDomain=network_engine_domain  SubClassName=ps_output  LeftPortType=input  RightPortType=output  PseudoPeriodic=off  Frequencies=[]  Unit=A  AffineConversion=off
  VBatt : PMIOPort  Side=Left
  IBatt : PMIOPort  Port=2  Side=Left
  Batt_Ah : Outport
  Batt_Meas : Outport  Port=2
  tag scope: Batt_Measures=global
  wires:
  Calculate battery power & charge/1(Ah) -> Bus Creator/1, Calc Pct/1, Batt_Ah/1  "Batt_Ah"
  Calc Pct/1 -> Bus Creator/2  "SOC (%)"
  PS-Simulink Converter1/1 -> Bus Creator/3  "Voltage (V)"
  PS-Simulink Converter2/1 -> Bus Creator/4  "Current (A)"
  Bus Creator/1 -> [Batt_Measures], Batt_Meas/1
  connections:
  Calculate battery power & charge/LConn1 -- VBatt/RConn1 -- PS-Simulink Converter1/LConn1
  Calculate battery power & charge/LConn2 -- IBatt/RConn1 -- PS-Simulink Converter2/LConn1

== system HEV_Battery_Lib_org/Predefined/GF1 ==
  In1 : Inport
  SOC Offset : Subsystem
      mask Display: disp('A')
  Out1 : Outport
  tag scope: Batt_Measures=global
  wires:
  SOC Offset/1(Out1) -> Out1/1, [Batt_Measures]
  In1/1 -> SOC Offset/1(In1)

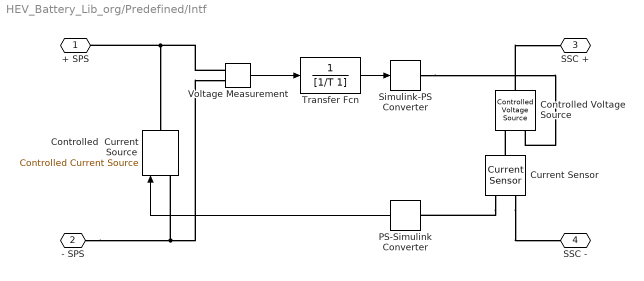
== system HEV_Battery_Lib_org/Predefined/Intf ==
  Controlled Voltage Source : fl_lib/Electrical/Electrical Sources/Controlled Voltage Source
  Controlled  Current Source : powerlib/Electrical Sources/Controlled Current Source  Initialize=on  Source_Type=AC  Amplitude=0  Phase=0  Frequency=0  Measurements=None
      settings: SourceProductName=Simscape Electrical
  Current Sensor : fl_lib/Electrical/Electrical Sensors/Current Sensor
  PS-Simulink Converter : nesl_utility/PS-Simulink Converter  PhysicalDomain=network_engine_domain  SubClassName=ps_output  LeftPortType=input  RightPortType=output  PseudoPeriodic=off  Frequencies=[]  Unit=A  AffineConversion=off
  Simulink-PS Converter : nesl_utility/Simulink-PS Converter  PhysicalDomain=network_engine_domain  SubClassName=ps_input  LeftPortType=input  RightPortType=output  PseudoPeriodic=off  Frequencies=[]  NoiseDistribution=none  NoiseParameters=[]  Unit=V  AffineConversion=off  FilteringAndDerivatives=zero  SimscapeFilterOrder=1  InputFilterTimeConstant=.001  UdotUserProvided=0
  Transfer Fcn : TransferFcn  Denominator=[1/T 1]
  Voltage Measurement : powerlib/Measurements/Voltage Measurement  PhasorSimulation=off  OutputType=Complex  PSBequivalent=0
      settings: SourceProductName=Simscape Electrical
  + SPS : PMIOPort  Side=Left
  - SPS : PMIOPort  Port=2  Side=Left
  SSC + : PMIOPort  Port=3  Side=Right
  SSC - : PMIOPort  Port=4  Side=Right
  wires:
  Transfer Fcn/1 -> Simulink-PS Converter/1
  Voltage Measurement/1 -> Transfer Fcn/1
  PS-Simulink Converter/1 -> Controlled  Current Source/1
  connections:
  Voltage Measurement/LConn1 -- + SPS/RConn1 -- Controlled  Current Source/RConn1
  Current Sensor/RConn2 -- SSC -/RConn1
  - SPS/RConn1 -- Voltage Measurement/LConn2 -- Controlled  Current Source/LConn1
  Current Sensor/RConn1 -- PS-Simulink Converter/LConn1
  Simulink-PS Converter/RConn1 -- Controlled Voltage Source/RConn1
  Current Sensor/LConn1 -- Controlled Voltage Source/RConn2
  Controlled Voltage Source/LConn1 -- SSC +/RConn1

== system HEV_Battery_Lib_org/RCGeneric/Measurements ==
  Bus Creator : BusCreator  Inputs=4
  Calc Pct : Gain  Gain=1/HEV_Param.Battery_Sys.Maximum_Capacity*100
  Calculate battery power & charge : Subsystem
  PS-Simulink Converter1 : nesl_utility/PS-Simulink Converter  PhysicalDomain=network_engine_domain  SubClassName=ps_output  LeftPortType=input  RightPortType=output  PseudoPeriodic=off  Frequencies=[]  Unit=V  AffineConversion=off
  PS-Simulink Converter2 : nesl_utility/PS-Simulink Converter  PhysicalDomain=network_engine_domain  SubClassName=ps_output  LeftPortType=input  RightPortType=output  PseudoPeriodic=off  Frequencies=[]  Unit=A  AffineConversion=off
  VBatt : PMIOPort  Side=Left
  IBatt : PMIOPort  Port=2  Side=Left
  Batt_Ah : Outport
  Batt_Meas : Outport  Port=2
  tag scope: Batt_Measures=global
  wires:
  Bus Creator/1 -> Batt_Meas/1, [Batt_Measures]
  PS-Simulink Converter2/1 -> Bus Creator/4  "Current (A)"
  PS-Simulink Converter1/1 -> Bus Creator/3  "Voltage (V)"
  Calc Pct/1 -> Bus Creator/2  "SOC (%)"
  Calculate battery power & charge/1(Ah) -> Batt_Ah/1, Calc Pct/1, Bus Creator/1  "Batt_Ah"
  connections:
  PS-Simulink Converter2/LConn1 -- IBatt/RConn1 -- Calculate battery power & charge/LConn2
  PS-Simulink Converter1/LConn1 -- VBatt/RConn1 -- Calculate battery power & charge/LConn1

== system HEV_Battery_Lib_org/Cells/Battery cell1/ DOC  ==
  PS-Simulink Converter1 : nesl_utility/PS-Simulink Converter  PhysicalDomain=network_engine_domain  SubClassName=ps_output  LeftPortType=input  RightPortType=output  PseudoPeriodic=off  Frequencies=[]  Unit=1  AffineConversion=off
  PS : PMIOPort  Side=Left
  tag scope: DOC=global
  wires:
  PS-Simulink Converter1/1 -> [DOC]
  connections:
  PS/RConn1 -- PS-Simulink Converter1/LConn1

== system HEV_Battery_Lib_org/Cells/Battery cell1/ SOC  ==
  PS-Simulink Converter1 : nesl_utility/PS-Simulink Converter  PhysicalDomain=network_engine_domain  SubClassName=ps_output  LeftPortType=input  RightPortType=output  PseudoPeriodic=off  Frequencies=[]  Unit=1  AffineConversion=off
  PS : PMIOPort  Side=Left
  tag scope: SOC=global
  wires:
  PS-Simulink Converter1/1 -> [SOC]
  connections:
  PS/RConn1 -- PS-Simulink Converter1/LConn1

== system HEV_Battery_Lib_org/Cells/Battery cell1/T ==
  PS-Simulink Converter1 : nesl_utility/PS-Simulink Converter  PhysicalDomain=network_engine_domain  SubClassName=ps_output  LeftPortType=input  RightPortType=output  PseudoPeriodic=off  Frequencies=[]  Unit=degC  AffineConversion=on
  PS : PMIOPort  Side=Left
  tag scope: Batt_Cell_Temp=global
  wires:
  PS-Simulink Converter1/1 -> [Batt_Cell_Temp]
  connections:
  PS/RConn1 -- PS-Simulink Converter1/LConn1

== system HEV_Battery_Lib_org/Cells/Battery cell1/Thermal Model ==
  Battery thermal mass : fl_lib/Thermal/Thermal Elements/Thermal Mass  mass=1 kg  sp_heat=HEV_Param.Battery_Cell.Ctheta J/kg/K  T_specify=on  T_priority=High  T=HEV_Param.Battery_Cell.theta_init+273 K  T_nominal_specify=off  T_nominal_unit=K  T_nominal_value=1  Q_specify=off  Q_priority=High  Q=0 J/s  Q_nominal_specify=off  Q_nominal_unit=J/s  Q_nominal_value=1
  Ideal Temperature Sensor : fl_lib/Thermal/Thermal Sensors/Ideal Temperature Sensor
      settings: SourceProductName=Simscape  SourceProductBaseCode=SS
  Ideal Heat Flow Source : fl_lib/Thermal/Thermal Sources/Ideal Heat Flow Source
      settings: SourceProductName=Simscape  SourceProductBaseCode=SS
  Kt as a function of temperature : fl_lib/Physical Signals/Lookup Tables/PS Lookup Table (1D)  x=[HEV_Param.Battery_Cell.theta_f,HEV_Param.Battery_Cell. Kt_Temps]+273  f=[0 HEV_Param.Battery_Cell.Kt]  interp_method=1  extrap_method=1
      settings: SourceProductName=Simscape  SourceProductBaseCode=SS
  Thermal Reference1 : fl_lib/Thermal/Thermal Elements/Thermal Reference
  Thermal Reference2 : fl_lib/Thermal/Thermal Elements/Thermal Reference
  Ps : PMIOPort  Tag=PMCPort  Side=Left
  H : PMIOPort  Tag=PMCPort  Port=2  Side=Left
  Kt : PMIOPort  Tag=PMCPort  Port=3  Side=Right
  T : PMIOPort  Tag=PMCPort  Port=4  Side=Right
  connections:
  Ideal Heat Flow Source/RConn1 -- Ps/RConn1
  Kt/RConn1 -- Kt as a function of temperature/RConn1
  Battery thermal mass/LConn1 -- Ideal Heat Flow Source/LConn1 -- Ideal Temperature Sensor/LConn1 -- H/RConn1
  Thermal Reference1/LConn1 -- Ideal Heat Flow Source/RConn2
  T/RConn1 -- Kt as a function of temperature/LConn1 -- Ideal Temperature Sensor/RConn2
  Ideal Temperature Sensor/RConn1 -- Thermal Reference2/LConn1

== system HEV_Battery_Lib_org/Cells/Battery cell2/Thermal Model ==
  Battery thermal mass : fl_lib/Thermal/Thermal Elements/Thermal Mass  mass=1 kg  sp_heat=HEV_Param.Battery_Cell.Ctheta J/kg/K  T_specify=on  T_priority=High  T=HEV_Param.Battery_Cell.theta_init+273 K  T_nominal_specify=off  T_nominal_unit=K  T_nominal_value=1  Q_specify=off  Q_priority=High  Q=0 J/s  Q_nominal_specify=off  Q_nominal_unit=J/s  Q_nominal_value=1
  Ideal Temperature Sensor : fl_lib/Thermal/Thermal Sensors/Ideal Temperature Sensor
      settings: SourceProductName=Simscape  SourceProductBaseCode=SS
  Ideal Heat Flow Source : fl_lib/Thermal/Thermal Sources/Ideal Heat Flow Source
      settings: SourceProductName=Simscape  SourceProductBaseCode=SS
  Kt as a function of temperature : fl_lib/Physical Signals/Lookup Tables/PS Lookup Table (1D)  x=[HEV_Param.Battery_Cell.theta_f,HEV_Param.Battery_Cell. Kt_Temps]+273  f=[0 HEV_Param.Battery_Cell.Kt]  interp_method=1  extrap_method=1
      settings: SourceProductName=Simscape  SourceProductBaseCode=SS
  Thermal Reference1 : fl_lib/Thermal/Thermal Elements/Thermal Reference
  Thermal Reference2 : fl_lib/Thermal/Thermal Elements/Thermal Reference
  Ps : PMIOPort  Tag=PMCPort  Side=Left
  H : PMIOPort  Tag=PMCPort  Port=2  Side=Left
  Kt : PMIOPort  Tag=PMCPort  Port=3  Side=Right
  T : PMIOPort  Tag=PMCPort  Port=4  Side=Right
  connections:
  Ideal Temperature Sensor/RConn1 -- Thermal Reference2/LConn1
  Ideal Temperature Sensor/RConn2 -- Kt as a function of temperature/LConn1 -- T/RConn1
  Thermal Reference1/LConn1 -- Ideal Heat Flow Source/RConn2
  H/RConn1 -- Ideal Temperature Sensor/LConn1 -- Ideal Heat Flow Source/LConn1 -- Battery thermal mass/LConn1
  Kt/RConn1 -- Kt as a function of temperature/RConn1
  Ideal Heat Flow Source/RConn1 -- Ps/RConn1

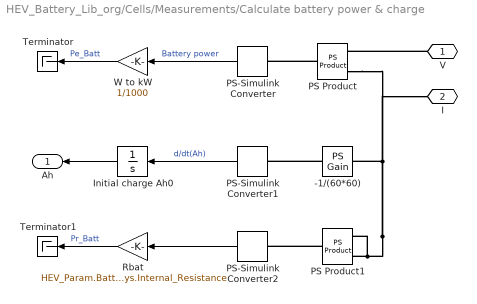
== system HEV_Battery_Lib_org/Cells/Measurements/Calculate battery power & charge ==
  -1/(60*60) : fl_lib/Physical Signals/Functions/PS Gain  gain=-1/(60*60)
  Initial charge Ah0 : Integrator  InitialCondition=HEV_Param.Battery_Sys.Maximum_Capacity
  PS Product : fl_lib/Physical Signals/Functions/PS Product
      settings: SourceProductName=Simscape
  PS Product1 : fl_lib/Physical Signals/Functions/PS Product
      settings: SourceProductName=Simscape
  PS-Simulink Converter : nesl_utility/PS-Simulink Converter  PhysicalDomain=network_engine_domain  SubClassName=ps_output  LeftPortType=input  RightPortType=output  PseudoPeriodic=off  Frequencies=[]  Unit=W  AffineConversion=off
  PS-Simulink Converter1 : nesl_utility/PS-Simulink Converter  PhysicalDomain=network_engine_domain  SubClassName=ps_output  LeftPortType=input  RightPortType=output  PseudoPeriodic=off  Frequencies=[]  Unit=1  AffineConversion=off
  PS-Simulink Converter2 : nesl_utility/PS-Simulink Converter  PhysicalDomain=network_engine_domain  SubClassName=ps_output  LeftPortType=input  RightPortType=output  PseudoPeriodic=off  Frequencies=[]  Unit=1  AffineConversion=off
  Rbat : Gain  Gain=HEV_Param.Battery_Sys.Internal_Resistance
  Terminator : Terminator
  Terminator1 : Terminator
  W to kW : Gain  Gain=1/1000
  V : PMIOPort  Side=Left
  I : PMIOPort  Port=2  Side=Left
  Ah : Outport
  wires:
  Rbat/1 -> Terminator1/1  "Pr_Batt"
  PS-Simulink Converter2/1 -> Rbat/1
  Initial charge Ah0/1 -> Ah/1
  PS-Simulink Converter1/1 -> Initial charge Ah0/1  "d/dt(Ah)"
  W to kW/1 -> Terminator/1  "Pe_Batt"
  PS-Simulink Converter/1 -> W to kW/1  "Battery power"
  connections:
  PS Product1/RConn1 -- PS-Simulink Converter2/LConn1
  -1/(60*60)/RConn1 -- PS-Simulink Converter1/LConn1
  PS Product1/LConn2 -- PS Product1/LConn1 -- -1/(60*60)/LConn1 -- I/RConn1 -- PS Product/LConn2
  V/RConn1 -- PS Product/LConn1
  PS Product/RConn1 -- PS-Simulink Converter/LConn1

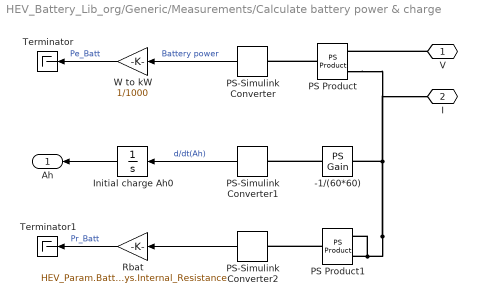
== system HEV_Battery_Lib_org/Generic/Measurements/Calculate battery power & charge ==
  -1/(60*60) : fl_ps_legacy_lib/Legacy Physical Signals/Functions/PS Gain  gain=-1/(60*60)
      settings: SourceProductName=Simscape
  Initial charge Ah0 : Integrator  InitialCondition=HEV_Param.Battery_Sys.Maximum_Capacity
  PS Product : fl_ps_legacy_lib/Legacy Physical Signals/Functions/PS Product
      settings: SourceProductName=Simscape  SourceProductBaseCode=SS
  PS Product1 : fl_ps_legacy_lib/Legacy Physical Signals/Functions/PS Product
      settings: SourceProductName=Simscape  SourceProductBaseCode=SS
  PS-Simulink Converter : nesl_utility/PS-Simulink Converter  PhysicalDomain=network_engine_domain  SubClassName=ps_output  LeftPortType=input  RightPortType=output  PseudoPeriodic=off  Frequencies=[]  Unit=W  AffineConversion=off
  PS-Simulink Converter1 : nesl_utility/PS-Simulink Converter  PhysicalDomain=network_engine_domain  SubClassName=ps_output  LeftPortType=input  RightPortType=output  PseudoPeriodic=off  Frequencies=[]  Unit=1  AffineConversion=off
  PS-Simulink Converter2 : nesl_utility/PS-Simulink Converter  PhysicalDomain=network_engine_domain  SubClassName=ps_output  LeftPortType=input  RightPortType=output  PseudoPeriodic=off  Frequencies=[]  Unit=1  AffineConversion=off
  Rbat : Gain  Gain=HEV_Param.Battery_Sys.Internal_Resistance
  Terminator : Terminator
  Terminator1 : Terminator
  W to kW : Gain  Gain=1/1000
  V : PMIOPort  Side=Left
  I : PMIOPort  Port=2  Side=Left
  Ah : Outport
  wires:
  Rbat/1 -> Terminator1/1  "Pr_Batt"
  PS-Simulink Converter2/1 -> Rbat/1
  Initial charge Ah0/1 -> Ah/1
  PS-Simulink Converter1/1 -> Initial charge Ah0/1  "d/dt(Ah)"
  W to kW/1 -> Terminator/1  "Pe_Batt"
  PS-Simulink Converter/1 -> W to kW/1  "Battery power"
  connections:
  PS Product1/RConn1 -- PS-Simulink Converter2/LConn1
  -1/(60*60)/RConn1 -- PS-Simulink Converter1/LConn1
  PS Product1/LConn2 -- PS Product1/LConn1 -- -1/(60*60)/LConn1 -- I/RConn1 -- PS Product/LConn2
  V/RConn1 -- PS Product/LConn1
  PS Product/RConn1 -- PS-Simulink Converter/LConn1

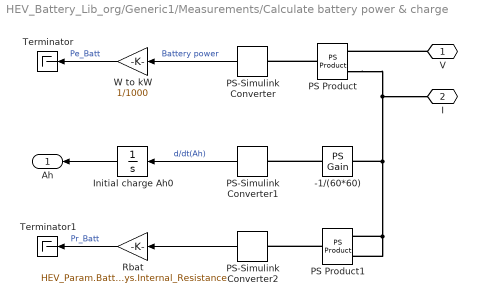
== system HEV_Battery_Lib_org/Generic1/Measurements/Calculate battery power & charge ==
  -1/(60*60) : fl_ps_legacy_lib/Legacy Physical Signals/Functions/PS Gain  gain=-1/(60*60)
      settings: SourceProductName=Simscape
  Initial charge Ah0 : Integrator  InitialCondition=HEV_Param.Battery_Sys.Maximum_Capacity
  PS Product : fl_ps_legacy_lib/Legacy Physical Signals/Functions/PS Product
      settings: SourceProductName=Simscape  SourceProductBaseCode=SS
  PS Product1 : fl_ps_legacy_lib/Legacy Physical Signals/Functions/PS Product
      settings: SourceProductName=Simscape  SourceProductBaseCode=SS
  PS-Simulink Converter : nesl_utility/PS-Simulink Converter  PhysicalDomain=network_engine_domain  SubClassName=ps_output  LeftPortType=input  RightPortType=output  PseudoPeriodic=off  Frequencies=[]  Unit=W  AffineConversion=off
  PS-Simulink Converter1 : nesl_utility/PS-Simulink Converter  PhysicalDomain=network_engine_domain  SubClassName=ps_output  LeftPortType=input  RightPortType=output  PseudoPeriodic=off  Frequencies=[]  Unit=1  AffineConversion=off
  PS-Simulink Converter2 : nesl_utility/PS-Simulink Converter  PhysicalDomain=network_engine_domain  SubClassName=ps_output  LeftPortType=input  RightPortType=output  PseudoPeriodic=off  Frequencies=[]  Unit=1  AffineConversion=off
  Rbat : Gain  Gain=HEV_Param.Battery_Sys.Internal_Resistance
  Terminator : Terminator
  Terminator1 : Terminator
  W to kW : Gain  Gain=1/1000
  V : PMIOPort  Side=Left
  I : PMIOPort  Port=2  Side=Left
  Ah : Outport
  wires:
  PS-Simulink Converter/1 -> W to kW/1  "Battery power"
  W to kW/1 -> Terminator/1  "Pe_Batt"
  PS-Simulink Converter1/1 -> Initial charge Ah0/1  "d/dt(Ah)"
  Initial charge Ah0/1 -> Ah/1
  PS-Simulink Converter2/1 -> Rbat/1
  Rbat/1 -> Terminator1/1  "Pr_Batt"
  connections:
  PS Product/RConn1 -- PS-Simulink Converter/LConn1
  V/RConn1 -- PS Product/LConn1
  PS Product/LConn2 -- I/RConn1 -- -1/(60*60)/LConn1 -- PS Product1/LConn1 -- PS Product1/LConn2
  -1/(60*60)/RConn1 -- PS-Simulink Converter1/LConn1
  PS Product1/RConn1 -- PS-Simulink Converter2/LConn1

== system HEV_Battery_Lib_org/Predefined/GF1/SOC Offset ==
  note: For control logic to work consistently
      | for all versions, SOC% must be scaled
  In1 : Inport
  Bus Creator : BusCreator  Inputs=4
  Bus Selector : BusSelector  OutputSignals=SOC (%)
  Bus Selector1 : BusSelector  OutputSignals=Current (A),Voltage (V)
  Gain : Gain  Gain=100/HEV_Param.Battery_Det.Initial_SOC
  Gain1 : Gain  Gain=-1/(60*60)
  Initial charge Ah0 : Integrator  InitialCondition=HEV_Param.Battery_Det.Rated_Capacity*HEV_Param.Battery_Det.Initial_SOC/100
  Out1 : Outport
  wires:
  In1/1 -> Bus Selector/1, Bus Selector1/1
  Bus Selector/1 -> Gain/1  "<SOC (%)>"
  Bus Selector1/1 -> Bus Creator/2, Gain1/1  "<Current (A)>"
  Gain/1 -> Bus Creator/4  "SOC (%)"
  Bus Selector1/2 -> Bus Creator/3  "<Voltage (V)>"
  Bus Creator/1 -> Out1/1
  Gain1/1 -> Initial charge Ah0/1
  Initial charge Ah0/1 -> Bus Creator/1  "Batt_Ah"

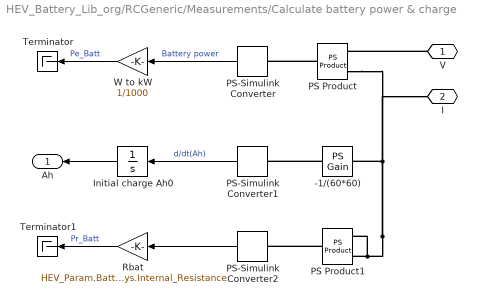
== system HEV_Battery_Lib_org/RCGeneric/Measurements/Calculate battery power & charge ==
  -1/(60*60) : fl_ps_legacy_lib/Legacy Physical Signals/Functions/PS Gain  gain=-1/(60*60)
      settings: SourceProductName=Simscape
  Initial charge Ah0 : Integrator  InitialCondition=HEV_Param.Battery_Sys.Maximum_Capacity
  PS Product : fl_ps_legacy_lib/Legacy Physical Signals/Functions/PS Product
      settings: SourceProductName=Simscape  SourceProductBaseCode=SS
  PS Product1 : fl_ps_legacy_lib/Legacy Physical Signals/Functions/PS Product
      settings: SourceProductName=Simscape  SourceProductBaseCode=SS
  PS-Simulink Converter : nesl_utility/PS-Simulink Converter  PhysicalDomain=network_engine_domain  SubClassName=ps_output  LeftPortType=input  RightPortType=output  PseudoPeriodic=off  Frequencies=[]  Unit=W  AffineConversion=off
  PS-Simulink Converter1 : nesl_utility/PS-Simulink Converter  PhysicalDomain=network_engine_domain  SubClassName=ps_output  LeftPortType=input  RightPortType=output  PseudoPeriodic=off  Frequencies=[]  Unit=1  AffineConversion=off
  PS-Simulink Converter2 : nesl_utility/PS-Simulink Converter  PhysicalDomain=network_engine_domain  SubClassName=ps_output  LeftPortType=input  RightPortType=output  PseudoPeriodic=off  Frequencies=[]  Unit=1  AffineConversion=off
  Rbat : Gain  Gain=HEV_Param.Battery_Sys.Internal_Resistance
  Terminator : Terminator
  Terminator1 : Terminator
  W to kW : Gain  Gain=1/1000
  V : PMIOPort  Side=Left
  I : PMIOPort  Port=2  Side=Left
  Ah : Outport
  wires:
  Rbat/1 -> Terminator1/1  "Pr_Batt"
  PS-Simulink Converter2/1 -> Rbat/1
  Initial charge Ah0/1 -> Ah/1
  PS-Simulink Converter1/1 -> Initial charge Ah0/1  "d/dt(Ah)"
  W to kW/1 -> Terminator/1  "Pe_Batt"
  PS-Simulink Converter/1 -> W to kW/1  "Battery power"
  connections:
  PS Product1/RConn1 -- PS-Simulink Converter2/LConn1
  -1/(60*60)/RConn1 -- PS-Simulink Converter1/LConn1
  PS Product1/LConn2 -- PS Product1/LConn1 -- -1/(60*60)/LConn1 -- I/RConn1 -- PS Product/LConn2
  V/RConn1 -- PS Product/LConn1
  PS Product/RConn1 -- PS-Simulink Converter/LConn1
